simulink model "LaneMergingSim"  (R2015a)
settings: Solver=ode3  StartTime=0.0  StopTime=11.0  FixedStep=0.1  RelTol=1e-3
libraries: simulink x1
settings Model: Creator=ppnathan  LastModifiedBy=ppnathan

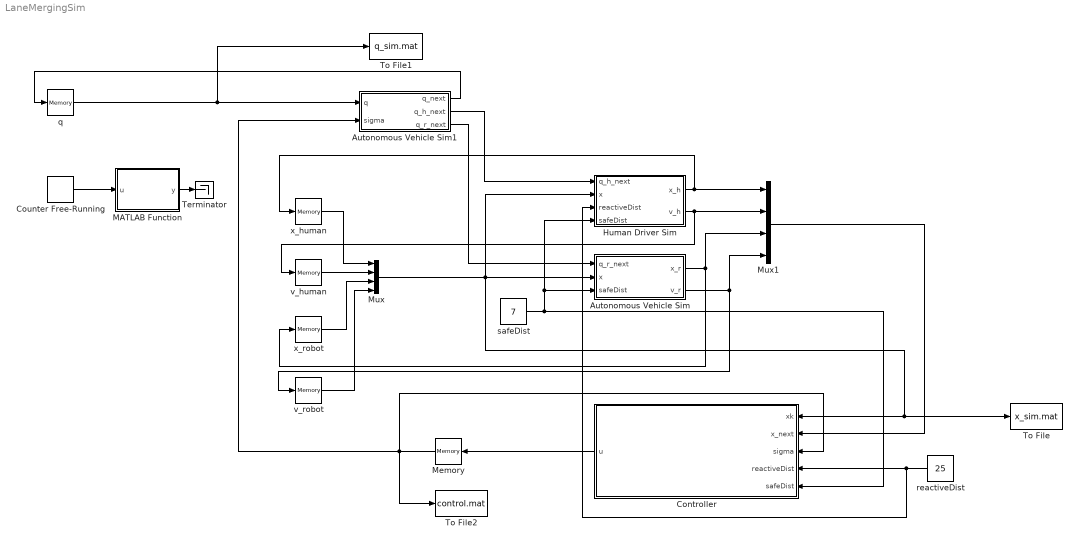
== system LaneMergingSim ==
  Autonomous Vehicle Sim : Subsystem
  Autonomous Vehicle Sim1 : Subsystem
  Controller : Subsystem
  Counter Free-Running : simulink/Sources/Counter Free-Running  NumBits=32  tsamp=-1
  Human Driver Sim : Subsystem
  MATLAB Function : MATLAB Function  TreatAsAtomicUnit=on
  Memory : Memory  X0=1  InheritSampleTime=on
  Mux : Mux
  Mux1 : Mux
  Terminator : Terminator
  To File : ToFile  Filename=x_sim.mat  MatrixName=x_sim
  To File1 : ToFile  Filename=q_sim.mat  MatrixName=q_sim
  To File2 : ToFile  Filename=control.mat  MatrixName=control
  q : Memory  X0=7  InheritSampleTime=on
  reactiveDist : Constant  Value=25
  safeDist : Constant  Value=7
  v_human : Memory  X0=30  InheritSampleTime=on
  v_robot : Memory  X0=32  InheritSampleTime=on
  x_human : Memory  X0=-300  InheritSampleTime=on
  x_robot : Memory  X0=-330  InheritSampleTime=on
  wires:
  x_human/1 -> Mux/1
  v_human/1 -> Mux/2
  x_robot/1 -> Mux/3
  v_robot/1 -> Mux/4
  Autonomous Vehicle Sim1/1(q_next) -> q/1
  Human Driver Sim/1(x_h) -> x_human/1, Mux1/1
  Human Driver Sim/2(v_h) -> Mux1/2, v_human/1
  Autonomous Vehicle Sim/1(x_r) -> Mux1/3, x_robot/1
  Autonomous Vehicle Sim/2(v_r) -> v_robot/1, Mux1/4
  Autonomous Vehicle Sim1/2(q_h_next) -> Human Driver Sim/1(q_h_next)
  Autonomous Vehicle Sim1/3(q_r_next) -> Autonomous Vehicle Sim/1(q_r_next)
  safeDist/1 -> Controller/5("safeDist "), Human Driver Sim/4(safeDist), Autonomous Vehicle Sim/3(safeDist)
  reactiveDist/1 -> Human Driver Sim/3(reactiveDist), Controller/4(reactiveDist)
  Mux1/1 -> Controller/2("x_next ")
  Controller/1(u) -> Memory/1
  Mux/1 -> To File/1, Controller/1(xk), Human Driver Sim/2(x), Autonomous Vehicle Sim/2(x)
  q/1 -> To File1/1, Autonomous Vehicle Sim1/1(q)
  Memory/1 -> Controller/3("sigma "), To File2/1, Autonomous Vehicle Sim1/2(sigma)
  Counter Free-Running/1 -> MATLAB Function/1(u)
  MATLAB Function/1(y) -> Terminator/1

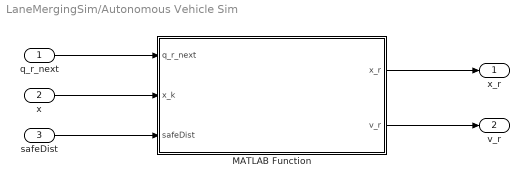
== system LaneMergingSim/Autonomous Vehicle Sim ==
  q_r_next : Inport
  x : Inport  Port=2  PortDimensions=4
  safeDist : Inport  Port=3
  MATLAB Function : MATLAB Function  TreatAsAtomicUnit=on
  x_r : Outport
  v_r : Outport  Port=2
  wires:
  MATLAB Function/1(x_r) -> x_r/1
  MATLAB Function/2(v_r) -> v_r/1
  x/1 -> MATLAB Function/2(x_k)
  q_r_next/1 -> MATLAB Function/1(q_r_next)
  safeDist/1 -> MATLAB Function/3(safeDist)

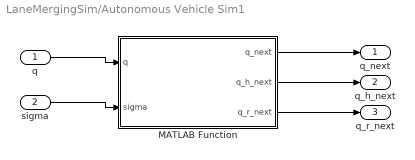
== system LaneMergingSim/Autonomous Vehicle Sim1 ==
  q : Inport
  sigma : Inport  Port=2
  MATLAB Function : MATLAB Function  TreatAsAtomicUnit=on
  q_next : Outport
  q_h_next : Outport  Port=2
  q_r_next : Outport  Port=3
  wires:
  q/1 -> MATLAB Function/1(q)
  sigma/1 -> MATLAB Function/2(sigma)
  MATLAB Function/2(q_h_next) -> q_h_next/1
  MATLAB Function/3(q_r_next) -> q_r_next/1
  MATLAB Function/1(q_next) -> q_next/1

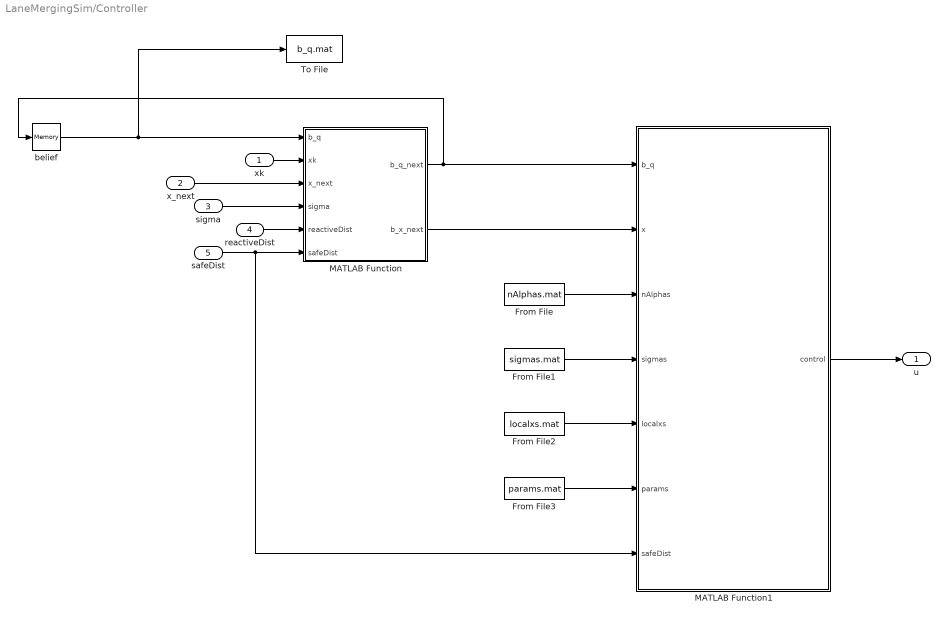
== system LaneMergingSim/Controller ==
  xk : Inport
  "x_next " : Inport  Port=2  PortDimensions=4
  "sigma " : Inport  Port=3
  reactiveDist : Inport  Port=4
  "safeDist " : Inport  Port=5
  From File : FromFile  FileName=nAlphas.mat
  From File1 : FromFile  FileName=sigmas.mat
  From File2 : FromFile  FileName=localxs.mat
  From File3 : FromFile  FileName=params.mat
  MATLAB Function : MATLAB Function  TreatAsAtomicUnit=on
  MATLAB Function1 : MATLAB Function  TreatAsAtomicUnit=on
  To File : ToFile  Filename=b_q.mat  MatrixName=b_q
  belief : Memory  X0="[0.25, 0, 0, 0.25, 0, 0,  0.25, 0, 0, 0.25, 0, 0]"
  u : Outport  PortDimensions=1
  wires:
  MATLAB Function/1(b_q_next) -> belief/1, MATLAB Function1/1(b_q)
  MATLAB Function/2(b_x_next) -> MATLAB Function1/2(x)
  From File/1 -> MATLAB Function1/3(nAlphas)
  From File1/1 -> MATLAB Function1/4(sigmas)
  From File2/1 -> MATLAB Function1/5(localxs)
  From File3/1 -> MATLAB Function1/6(params)
  "safeDist "/1 -> MATLAB Function1/7(safeDist), MATLAB Function/6(safeDist)
  MATLAB Function1/1(control) -> u/1
  reactiveDist/1 -> MATLAB Function/5(reactiveDist)
  xk/1 -> MATLAB Function/2(xk)
  "x_next "/1 -> MATLAB Function/3(x_next)
  "sigma "/1 -> MATLAB Function/4(sigma)
  belief/1 -> To File/1, MATLAB Function/1(b_q)

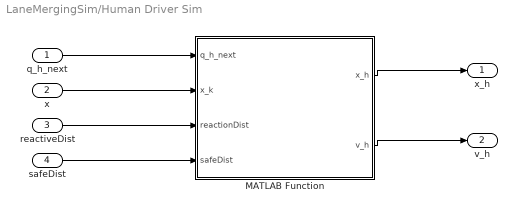
== system LaneMergingSim/Human Driver Sim ==
  q_h_next : Inport  PortDimensions=1
  x : Inport  Port=2  PortDimensions=4
  reactiveDist : Inport  Port=3  PortDimensions=1
  safeDist : Inport  Port=4
  MATLAB Function : MATLAB Function  TreatAsAtomicUnit=on
  x_h : Outport
  v_h : Outport  Port=2
  wires:
  x/1 -> MATLAB Function/2(x_k)
  q_h_next/1 -> MATLAB Function/1(q_h_next)
  MATLAB Function/1(x_h) -> x_h/1
  MATLAB Function/2(v_h) -> v_h/1
  safeDist/1 -> MATLAB Function/4(safeDist)
  reactiveDist/1 -> MATLAB Function/3(reactionDist)

== matlab function LaneMergingSim/Controller/MATLAB Function1 ==
  data: b_q input; control output; x input; nAlphas input; sigmas input; localxs input; params input; safeDist input
function control = FindOptimalContol(b_q, x, nAlphas, sigmas, localxs, params, safeDist)

nCState = length(x);
localxs = reshape(localxs, nCState, []);
params = reshape(params, 21, 12, []);
thresholddist = 10;
nDState = length(b_q);

bestvalue = -1e20;
bestidx = -1;

mindist = 1e20;
mindistidx = -1;

for n = 1:nAlphas
    sum  = 0;
    dist = norm(x - localxs(:, n));
    if (dist < thresholddist && (SatisfyConstraints(x, safeDist) || ...
		                         ~SatisfyConstraints(localxs(:, n), safeDist)))
        for q = 1:nDState
            const_term = params(1, q, n);
            first_order_term = params(2:(1+nCState), q, n);
            second_order_term = params((2+nCState):(1+nCState+nCState*nCState), q, n);
            second_order_term_reshape = reshape(second_order_term, nCState, nCState);
            sum = sum + b_q(q) * (const_term + first_order_term' * (x - localxs(:, n)) + ...
                                  (x - localxs(:, n))' * second_order_term_reshape * (x - localxs(:, n)));
        end
        
        if (sum > bestvalue)
            bestvalue = sum;
            bestidx = n;
        end
    end
    if (dist < mindist)
        mindist = dist;
        mindistidx = n;
    end
end

if (bestidx == -1)
    bestidx = mindistidx;
    disp('No point within the threshold, use policy with the nearest point.');
end

control = sigmas(bestidx);
disp('control = ');
disp(control);


end

== matlab function LaneMergingSim/Controller/MATLAB Function ==
  data: b_q input; b_q_next output; xk input; x_next input; sigma input; b_x_next output; reactiveDist input; safeDist input
function [b_q_next, b_x_next] = CalBelief(b_q, xk, x_next, sigma, reactiveDist, safeDist)

nDState = length(b_q);
b_q_next = zeros(nDState, 1);

if (norm(x_next - xk) < 1e-6)
    b_q_next = b_q;
else
    
    for qq = 1:nDState
        tmp = 0;
        for q = 1:nDState
            tmp = tmp + DStateTransfn(qq, q, sigma) * b_q(q);
        end
        b_q_next(qq) = DObsfn(0, qq) * ...
                       CStateTransfn(x_next, qq, xk, reactiveDist, safeDist) * tmp;
    end

    if (sum(b_q_next) == 0)
        b_q_next = b_q;
    else
        b_q_next = b_q_next / sum(b_q_next);
    end
end

b_x_next = x_next;

end

== matlab function LaneMergingSim/Human Driver Sim/MATLAB Function ==
  data: q_h_next input; x_h output; x_k input; reactionDist input; v_h output; safeDist input
function [x_h, v_h] = SampleHumanDriverState(q_h_next, x_k, reactionDist, safeDist)

if (~SatisfyConstraints(x_k, safeDist))
    x_h =  x_k(1);
    v_h =  x_k(2);
    
else
    OBLIVIOUS = 1; AGGRESSIVE = 2; COURTEOUS = 3; REASONABLE = 4;
    mNoiseMean = 0;
    mDistNoiseStd = 0.1;
    mVelNoiseStd = 0.1;
    mDeltaT = 0.1;

    humanDriver = q_h_next;

    if (humanDriver == OBLIVIOUS)
            humanInput = 0;
    elseif (humanDriver == AGGRESSIVE)
        if (abs(x_k(1) - x_k(3)) < reactionDist)
            humanInput = 1;
        else
            humanInput = 0;
        end
    elseif (humanDriver == COURTEOUS)
        if (abs(x_k(1) - x_k(3)) < reactionDist)
            humanInput = -1; 
        else
            humanInput = 0;
        end
    elseif (humanDriver == REASONABLE)
        if (abs(x_k(1) - x_k(3)) < reactionDist)
            if (x_k(2) > x_k(4))
                humanInput = 1;
            else
                humanInput = -1;
            end
        else
            humanInput = 0;
        end
    else
        humanInput = 0;
        disp('SampleHumanDriverState: q_next out of domain');
    end
    
    distNoise4HumanDriver = normrnd(mNoiseMean, mDistNoiseStd);
    velNoise4HumanDriver = normrnd(mNoiseMean, mVelNoiseStd);
    
    x_h = x_k(1) + mDeltaT * x_k(2) + distNoise4HumanDriver;
    v_h = x_k(2) + mDeltaT * humanInput + velNoise4HumanDriver;
end


end

== matlab function LaneMergingSim/Autonomous Vehicle Sim1/MATLAB Function ==
  data: q_next output; q input; q_h_next output; sigma input; q_r_next output
function [q_next, q_h_next, q_r_next] = SampleDState(q, sigma)

q_h_next = ceil(q / 3);

q_r_next = sigma;

q_next = (q_h_next - 1) * 3 + q_r_next;

end

== matlab function LaneMergingSim/Autonomous Vehicle Sim/MATLAB Function ==
  data: q_r_next input; x_r output; x_k input; safeDist input; v_r output
function [x_r, v_r] = SampleAutonomousVehicleState(q_r_next, x_k, safeDist)

if (~SatisfyConstraints(x_k, safeDist))
    x_r =  x_k(3);
    v_r =  x_k(4);
else
    mNoiseMean = 0;
    mDistNoiseStd = 0.1;
    mVelNoiseStd = 0.1;
    mDeltaT = 0.1;
    
    autonomousDriver = q_r_next;
    
    if (autonomousDriver == 1)
        autonomousInput = 0;
    elseif (autonomousDriver == 2)
        autonomousInput = 1;
    elseif (autonomousDriver == 3)
        autonomousInput = -1;
    else
        autonomousInput = 0;
        disp('SampleAutonomousVehicleState(): q_next out of domain');
    end
    
    distNoise4AutonomousDriver = normrnd(mNoiseMean, mDistNoiseStd);
    velNoise4AutonomousDriver = normrnd(mNoiseMean, mVelNoiseStd);
    
    x_r = x_k(3) + mDeltaT * x_k(4) + distNoise4AutonomousDriver;
    v_r = x_k(4) + mDeltaT * autonomousInput + velNoise4AutonomousDriver;
    
end

== matlab function LaneMergingSim/MATLAB Function ==
  data: u input; y output
function y = PrintCounts(u)
disp('count = ');
disp(u);

y = u;
